simulink model "ALL_JP360_DBW_V6_5_1103"  (R2022a)
settings: Solver=FixedStepAuto  StartTime=0.0  StopTime=inf  FixedStep=0.01  RelTol=1e-3  EnableMultiTasking=on
model workspace (MAT data in the model file):
  g = 9.8
undefined symbols (not defined in the file or in its folder): canChannel, delta_v_p, IPM_Line_C0, IPM_Line_C1, IPM_Line_C2, IPM_Line_C3, M, M_p, MRR_ObjDistX, MRR_ObjDistY, MRR_ObjFusionCamID, MRR_ObjFusionSig, MRR_ObjID, MRR_ObjRelVelX, MRR_ObjRelVelY, MRR_ObjType, MRR_ObjUpdFlg, none, obj_vaild, untracktime, V, videoinput
libraries: canfdmsglib x230, canfdlib x76, slpidlib x24, simulink x18, dspstat3 x14, ctrlSharedLib x1, simulink_extras x1, imaqlib x1, realtime_pacer_lib x1, dspvision x1, visionsinks x1
(part 41 of 55)

== system ALL_JP360_DBW_V6_5_1103/MsgFromCAN/Subsystem1/Subsystem17 ==
  VR_ADCU_MRR_ObjHeader_0x680FromOutData : Inport
  Bus Selector1 : BusSelector  OutputSignals=IPM_ObjBlockCounter_18,IPM_ObjDistX_18,IPM_ObjDistY_18,IPM_ObjID_18,IPM_ObjRelAccelX_18,IPM_ObjRelAccelY_18,IPM_ObjRelVelX_18,IPM_ObjRelVelY_18,IPM_ObjType_18,IPM_Object_Age_18,IPM_Object_Existence_Probability_18,IPM_Object_Heading_18,IPM_Object_Height_18,IPM_Object_Length_18,IPM_Object_Motion_Status_18,IPM_Object_Width_18
  Data Type Conversion{1..2,4,6,16..27} (16 alike) : DataTypeConversion  OutDataTypeStr=single  SaturateOnIntegerOverflow=off  RndMeth=Floor
  Mux1 : Mux  Inputs=16
  Out2 : Outport
  wires:
  Bus Selector1/12 -> Data Type Conversion27/1  "<IPM_Object_Heading_18>"
  Bus Selector1/10 -> Data Type Conversion25/1  "<IPM_Object_Age_18>"
  Bus Selector1/11 -> Data Type Conversion26/1  "<IPM_Object_Existence_Probability_18>"
  Bus Selector1/9 -> Data Type Conversion24/1  "<IPM_ObjType_18>"
  Bus Selector1/7 -> Data Type Conversion22/1  "<IPM_ObjRelVelX_18>"
  Bus Selector1/5 -> Data Type Conversion20/1  "<IPM_ObjRelAccelX_18>"
  Bus Selector1/4 -> Data Type Conversion19/1  "<IPM_ObjID_18>"
  Bus Selector1/8 -> Data Type Conversion23/1  "<IPM_ObjRelVelY_18>"
  Bus Selector1/6 -> Data Type Conversion21/1  "<IPM_ObjRelAccelY_18>"
  Bus Selector1/3 -> Data Type Conversion18/1  "<IPM_ObjDistY_18>"
  Mux1/1 -> Out2/1
  Bus Selector1/2 -> Data Type Conversion17/1  "<IPM_ObjDistX_18>"
  VR_ADCU_MRR_ObjHeader_0x680FromOutData/1 -> Bus Selector1/1
  Bus Selector1/1 -> Data Type Conversion16/1  "<IPM_ObjBlockCounter_18>"
  Data Type Conversion27/1 -> Mux1/12
  Data Type Conversion26/1 -> Mux1/11
  Data Type Conversion21/1 -> Mux1/6
  Data Type Conversion23/1 -> Mux1/8
  Data Type Conversion25/1 -> Mux1/10
  Data Type Conversion19/1 -> Mux1/4
  Data Type Conversion20/1 -> Mux1/5
  Data Type Conversion22/1 -> Mux1/7
  Data Type Conversion24/1 -> Mux1/9
  Data Type Conversion16/1 -> Mux1/1
  Data Type Conversion18/1 -> Mux1/3
  Data Type Conversion17/1 -> Mux1/2
  Bus Selector1/13 -> Data Type Conversion1/1  "<IPM_Object_Height_18>"
  Bus Selector1/14 -> Data Type Conversion2/1  "<IPM_Object_Length_18>"
  Bus Selector1/15 -> Data Type Conversion4/1  "<IPM_Object_Motion_Status_18>"
  Bus Selector1/16 -> Data Type Conversion6/1  "<IPM_Object_Width_18>"
  Data Type Conversion1/1 -> Mux1/13
  Data Type Conversion2/1 -> Mux1/14
  Data Type Conversion4/1 -> Mux1/15
  Data Type Conversion6/1 -> Mux1/16

== system ALL_JP360_DBW_V6_5_1103/MsgFromCAN/Subsystem1/Subsystem18 ==
  VR_ADCU_MRR_ObjHeader_0x680FromOutData : Inport
  Bus Selector1 : BusSelector  OutputSignals=IPM_ObjBlockCounter_16,IPM_ObjDistX_16,IPM_ObjDistY_16,IPM_ObjID_16,IPM_ObjRelAccelX_16,IPM_ObjRelAccelY_16,IPM_ObjRelVelX_16,IPM_ObjRelVelY_16,IPM_ObjType_16,IPM_Object_Age_16,IPM_Object_Existence_Probability_16,IPM_Object_Heading_16,IPM_Object_Height_16,IPM_Object_Length_16,IPM_Object_Motion_Status_16,IPM_Object_Width_16
  Data Type Conversion{1..2,4,6,16..27} (16 alike) : DataTypeConversion  OutDataTypeStr=single  SaturateOnIntegerOverflow=off  RndMeth=Floor
  Mux1 : Mux  Inputs=16
  Out2 : Outport
  wires:
  Bus Selector1/12 -> Data Type Conversion27/1  "<IPM_Object_Heading_16>"
  Bus Selector1/10 -> Data Type Conversion25/1  "<IPM_Object_Age_16>"
  Bus Selector1/11 -> Data Type Conversion26/1  "<IPM_Object_Existence_Probability_16>"
  Bus Selector1/9 -> Data Type Conversion24/1  "<IPM_ObjType_16>"
  Bus Selector1/7 -> Data Type Conversion22/1  "<IPM_ObjRelVelX_16>"
  Bus Selector1/5 -> Data Type Conversion20/1  "<IPM_ObjRelAccelX_16>"
  Bus Selector1/4 -> Data Type Conversion19/1  "<IPM_ObjID_16>"
  Bus Selector1/8 -> Data Type Conversion23/1  "<IPM_ObjRelVelY_16>"
  Bus Selector1/6 -> Data Type Conversion21/1  "<IPM_ObjRelAccelY_16>"
  Bus Selector1/3 -> Data Type Conversion18/1  "<IPM_ObjDistY_16>"
  Mux1/1 -> Out2/1
  Bus Selector1/2 -> Data Type Conversion17/1  "<IPM_ObjDistX_16>"
  VR_ADCU_MRR_ObjHeader_0x680FromOutData/1 -> Bus Selector1/1
  Bus Selector1/1 -> Data Type Conversion16/1  "<IPM_ObjBlockCounter_16>"
  Data Type Conversion27/1 -> Mux1/12
  Data Type Conversion26/1 -> Mux1/11
  Data Type Conversion21/1 -> Mux1/6
  Data Type Conversion23/1 -> Mux1/8
  Data Type Conversion25/1 -> Mux1/10
  Data Type Conversion19/1 -> Mux1/4
  Data Type Conversion20/1 -> Mux1/5
  Data Type Conversion22/1 -> Mux1/7
  Data Type Conversion24/1 -> Mux1/9
  Data Type Conversion16/1 -> Mux1/1
  Data Type Conversion18/1 -> Mux1/3
  Data Type Conversion17/1 -> Mux1/2
  Bus Selector1/13 -> Data Type Conversion1/1  "<IPM_Object_Height_16>"
  Bus Selector1/14 -> Data Type Conversion2/1  "<IPM_Object_Length_16>"
  Bus Selector1/15 -> Data Type Conversion4/1  "<IPM_Object_Motion_Status_16>"
  Bus Selector1/16 -> Data Type Conversion6/1  "<IPM_Object_Width_16>"
  Data Type Conversion1/1 -> Mux1/13
  Data Type Conversion2/1 -> Mux1/14
  Data Type Conversion4/1 -> Mux1/15
  Data Type Conversion6/1 -> Mux1/16

== system ALL_JP360_DBW_V6_5_1103/MsgFromCAN/Subsystem1/Subsystem19 ==
  VR_ADCU_MRR_ObjHeader_0x680FromOutData : Inport
  Bus Selector1 : BusSelector  OutputSignals=IPM_ObjBlockCounter_19,IPM_ObjDistX_19,IPM_ObjDistY_19,IPM_ObjID_19,IPM_ObjRelAccelX_19,IPM_ObjRelAccelY_19,IPM_ObjRelVelX_19,IPM_ObjRelVelY_19,IPM_ObjType_19,IPM_Object_Age_19,IPM_Object_Existence_Probability_19,IPM_Object_Heading_19,IPM_Object_Height_19,IPM_Object_Length_19,IPM_Object_Motion_Status_19,IPM_Object_Width_19
  Data Type Conversion{1..2,4,6,16..27} (16 alike) : DataTypeConversion  OutDataTypeStr=single  SaturateOnIntegerOverflow=off  RndMeth=Floor
  Mux1 : Mux  Inputs=16
  Out2 : Outport
  wires:
  Data Type Conversion6/1 -> Mux1/16
  Data Type Conversion4/1 -> Mux1/15
  Data Type Conversion2/1 -> Mux1/14
  Data Type Conversion1/1 -> Mux1/13
  Bus Selector1/16 -> Data Type Conversion6/1  "<IPM_Object_Width_19>"
  Bus Selector1/15 -> Data Type Conversion4/1  "<IPM_Object_Motion_Status_19>"
  Bus Selector1/14 -> Data Type Conversion2/1  "<IPM_Object_Length_19>"
  Bus Selector1/13 -> Data Type Conversion1/1  "<IPM_Object_Height_19>"
  Data Type Conversion17/1 -> Mux1/2
  Data Type Conversion18/1 -> Mux1/3
  Data Type Conversion16/1 -> Mux1/1
  Data Type Conversion24/1 -> Mux1/9
  Data Type Conversion22/1 -> Mux1/7
  Data Type Conversion20/1 -> Mux1/5
  Data Type Conversion19/1 -> Mux1/4
  Data Type Conversion25/1 -> Mux1/10
  Data Type Conversion23/1 -> Mux1/8
  Data Type Conversion21/1 -> Mux1/6
  Data Type Conversion26/1 -> Mux1/11
  Data Type Conversion27/1 -> Mux1/12
  Bus Selector1/1 -> Data Type Conversion16/1  "<IPM_ObjBlockCounter_19>"
  VR_ADCU_MRR_ObjHeader_0x680FromOutData/1 -> Bus Selector1/1
  Bus Selector1/2 -> Data Type Conversion17/1  "<IPM_ObjDistX_19>"
  Mux1/1 -> Out2/1
  Bus Selector1/3 -> Data Type Conversion18/1  "<IPM_ObjDistY_19>"
  Bus Selector1/6 -> Data Type Conversion21/1  "<IPM_ObjRelAccelY_19>"
  Bus Selector1/8 -> Data Type Conversion23/1  "<IPM_ObjRelVelY_19>"
  Bus Selector1/4 -> Data Type Conversion19/1  "<IPM_ObjID_19>"
  Bus Selector1/5 -> Data Type Conversion20/1  "<IPM_ObjRelAccelX_19>"
  Bus Selector1/7 -> Data Type Conversion22/1  "<IPM_ObjRelVelX_19>"
  Bus Selector1/9 -> Data Type Conversion24/1  "<IPM_ObjType_19>"
  Bus Selector1/11 -> Data Type Conversion26/1  "<IPM_Object_Existence_Probability_19>"
  Bus Selector1/10 -> Data Type Conversion25/1  "<IPM_Object_Age_19>"
  Bus Selector1/12 -> Data Type Conversion27/1  "<IPM_Object_Heading_19>"

== system ALL_JP360_DBW_V6_5_1103/MsgFromCAN/Subsystem1/Subsystem2 ==
  VR_ADCU_MRR_ObjHeader_0x680FromOutData : Inport
  Bus Selector1 : BusSelector  OutputSignals=IPM_ObjBlockCounter_03,IPM_ObjDistX_03,IPM_ObjDistY_03,IPM_ObjID_03,IPM_ObjRelAccelX_03,IPM_ObjRelAccelY_03,IPM_ObjRelVelX_03,IPM_ObjRelVelY_03,IPM_ObjType_03,IPM_Object_Age_03,IPM_Object_Existence_Probability_03,IPM_Object_Heading_03,IPM_Object_Height_03,IPM_Object_Length_03,IPM_Object_Motion_Status_03,IPM_Object_Width_03
  Data Type Conversion{1..2,4,6,16..27} (16 alike) : DataTypeConversion  OutDataTypeStr=single  SaturateOnIntegerOverflow=off  RndMeth=Floor
  Mux1 : Mux  Inputs=16
  Out2 : Outport
  wires:
  Bus Selector1/12 -> Data Type Conversion27/1  "<IPM_Object_Heading_03>"
  Bus Selector1/10 -> Data Type Conversion25/1  "<IPM_Object_Age_03>"
  Bus Selector1/11 -> Data Type Conversion26/1  "<IPM_Object_Existence_Probability_03>"
  Bus Selector1/9 -> Data Type Conversion24/1  "<IPM_ObjType_03>"
  Bus Selector1/7 -> Data Type Conversion22/1  "<IPM_ObjRelVelX_03>"
  Bus Selector1/5 -> Data Type Conversion20/1  "<IPM_ObjRelAccelX_03>"
  Bus Selector1/4 -> Data Type Conversion19/1  "<IPM_ObjID_03>"
  Bus Selector1/8 -> Data Type Conversion23/1  "<IPM_ObjRelVelY_03>"
  Bus Selector1/6 -> Data Type Conversion21/1  "<IPM_ObjRelAccelY_03>"
  Bus Selector1/3 -> Data Type Conversion18/1  "<IPM_ObjDistY_03>"
  Mux1/1 -> Out2/1
  Bus Selector1/2 -> Data Type Conversion17/1  "<IPM_ObjDistX_03>"
  VR_ADCU_MRR_ObjHeader_0x680FromOutData/1 -> Bus Selector1/1
  Bus Selector1/1 -> Data Type Conversion16/1  "<IPM_ObjBlockCounter_03>"
  Data Type Conversion27/1 -> Mux1/12
  Data Type Conversion26/1 -> Mux1/11
  Data Type Conversion21/1 -> Mux1/6
  Data Type Conversion23/1 -> Mux1/8
  Data Type Conversion25/1 -> Mux1/10
  Data Type Conversion19/1 -> Mux1/4
  Data Type Conversion20/1 -> Mux1/5
  Data Type Conversion22/1 -> Mux1/7
  Data Type Conversion24/1 -> Mux1/9
  Data Type Conversion16/1 -> Mux1/1
  Data Type Conversion18/1 -> Mux1/3
  Data Type Conversion17/1 -> Mux1/2
  Bus Selector1/13 -> Data Type Conversion1/1  "<IPM_Object_Height_03>"
  Bus Selector1/14 -> Data Type Conversion2/1  "<IPM_Object_Length_03>"
  Bus Selector1/15 -> Data Type Conversion4/1  "<IPM_Object_Motion_Status_03>"
  Bus Selector1/16 -> Data Type Conversion6/1  "<IPM_Object_Width_03>"
  Data Type Conversion1/1 -> Mux1/13
  Data Type Conversion2/1 -> Mux1/14
  Data Type Conversion4/1 -> Mux1/15
  Data Type Conversion6/1 -> Mux1/16

== system ALL_JP360_DBW_V6_5_1103/MsgFromCAN/Subsystem1/Subsystem20 ==
  VR_ADCU_MRR_ObjHeader_0x680FromOutData : Inport
  Bus Selector1 : BusSelector  OutputSignals=IPM_ObjBlockCounter_20,IPM_ObjDistX_20,IPM_ObjDistY_20,IPM_ObjID_20,IPM_ObjRelAccelX_20,IPM_ObjRelAccelY_20,IPM_ObjRelVelX_20,IPM_ObjRelVelY_20,IPM_ObjType_20,IPM_Object_Age_20,IPM_Object_Existence_Probability_20,IPM_Object_Heading_20,IPM_Object_Height_20,IPM_Object_Length_20,IPM_Object_Motion_Status_20,IPM_Object_Width_20
  Data Type Conversion{1..2,4,6,16..27} (16 alike) : DataTypeConversion  OutDataTypeStr=single  SaturateOnIntegerOverflow=off  RndMeth=Floor
  Mux1 : Mux  Inputs=16
  Out2 : Outport
  wires:
  Bus Selector1/12 -> Data Type Conversion27/1  "<IPM_Object_Heading_20>"
  Bus Selector1/10 -> Data Type Conversion25/1  "<IPM_Object_Age_20>"
  Bus Selector1/11 -> Data Type Conversion26/1  "<IPM_Object_Existence_Probability_20>"
  Bus Selector1/9 -> Data Type Conversion24/1  "<IPM_ObjType_20>"
  Bus Selector1/7 -> Data Type Conversion22/1  "<IPM_ObjRelVelX_20>"
  Bus Selector1/5 -> Data Type Conversion20/1  "<IPM_ObjRelAccelX_20>"
  Bus Selector1/4 -> Data Type Conversion19/1  "<IPM_ObjID_20>"
  Bus Selector1/8 -> Data Type Conversion23/1  "<IPM_ObjRelVelY_20>"
  Bus Selector1/6 -> Data Type Conversion21/1  "<IPM_ObjRelAccelY_20>"
  Bus Selector1/3 -> Data Type Conversion18/1  "<IPM_ObjDistY_20>"
  Mux1/1 -> Out2/1
  Bus Selector1/2 -> Data Type Conversion17/1  "<IPM_ObjDistX_20>"
  VR_ADCU_MRR_ObjHeader_0x680FromOutData/1 -> Bus Selector1/1
  Bus Selector1/1 -> Data Type Conversion16/1  "<IPM_ObjBlockCounter_20>"
  Data Type Conversion27/1 -> Mux1/12
  Data Type Conversion26/1 -> Mux1/11
  Data Type Conversion21/1 -> Mux1/6
  Data Type Conversion23/1 -> Mux1/8
  Data Type Conversion25/1 -> Mux1/10
  Data Type Conversion19/1 -> Mux1/4
  Data Type Conversion20/1 -> Mux1/5
  Data Type Conversion22/1 -> Mux1/7
  Data Type Conversion24/1 -> Mux1/9
  Data Type Conversion16/1 -> Mux1/1
  Data Type Conversion18/1 -> Mux1/3
  Data Type Conversion17/1 -> Mux1/2
  Bus Selector1/13 -> Data Type Conversion1/1  "<IPM_Object_Height_20>"
  Bus Selector1/14 -> Data Type Conversion2/1  "<IPM_Object_Length_20>"
  Bus Selector1/15 -> Data Type Conversion4/1  "<IPM_Object_Motion_Status_20>"
  Bus Selector1/16 -> Data Type Conversion6/1  "<IPM_Object_Width_20>"
  Data Type Conversion1/1 -> Mux1/13
  Data Type Conversion2/1 -> Mux1/14
  Data Type Conversion4/1 -> Mux1/15
  Data Type Conversion6/1 -> Mux1/16

== system ALL_JP360_DBW_V6_5_1103/MsgFromCAN/Subsystem1/Subsystem3 ==
  VR_ADCU_MRR_ObjHeader_0x680FromOutData : Inport
  Bus Selector1 : BusSelector  OutputSignals=IPM_ObjBlockCounter_05,IPM_ObjDistX_05,IPM_ObjDistY_05,IPM_ObjID_05,IPM_ObjRelAccelX_05,IPM_ObjRelAccelY_05,IPM_ObjRelVelX_05,IPM_ObjRelVelY_05,IPM_ObjType_05,IPM_Object_Age_05,IPM_Object_Existence_Probability_05,IPM_Object_Heading_05,IPM_Object_Height_05,IPM_Object_Length_05,IPM_Object_Motion_Status_05,IPM_Object_Width_05
  Data Type Conversion{1..2,4,6,16..27} (16 alike) : DataTypeConversion  OutDataTypeStr=single  SaturateOnIntegerOverflow=off  RndMeth=Floor
  Mux1 : Mux  Inputs=16
  Out2 : Outport
  wires:
  Data Type Conversion6/1 -> Mux1/16
  Data Type Conversion4/1 -> Mux1/15
  Data Type Conversion2/1 -> Mux1/14
  Data Type Conversion1/1 -> Mux1/13
  Bus Selector1/16 -> Data Type Conversion6/1  "<IPM_Object_Width_05>"
  Bus Selector1/15 -> Data Type Conversion4/1  "<IPM_Object_Motion_Status_05>"
  Bus Selector1/14 -> Data Type Conversion2/1  "<IPM_Object_Length_05>"
  Bus Selector1/13 -> Data Type Conversion1/1  "<IPM_Object_Height_05>"
  Data Type Conversion17/1 -> Mux1/2
  Data Type Conversion18/1 -> Mux1/3
  Data Type Conversion16/1 -> Mux1/1
  Data Type Conversion24/1 -> Mux1/9
  Data Type Conversion22/1 -> Mux1/7
  Data Type Conversion20/1 -> Mux1/5
  Data Type Conversion19/1 -> Mux1/4
  Data Type Conversion25/1 -> Mux1/10
  Data Type Conversion23/1 -> Mux1/8
  Data Type Conversion21/1 -> Mux1/6
  Data Type Conversion26/1 -> Mux1/11
  Data Type Conversion27/1 -> Mux1/12
  Bus Selector1/1 -> Data Type Conversion16/1  "<IPM_ObjBlockCounter_05>"
  VR_ADCU_MRR_ObjHeader_0x680FromOutData/1 -> Bus Selector1/1
  Bus Selector1/2 -> Data Type Conversion17/1  "<IPM_ObjDistX_05>"
  Mux1/1 -> Out2/1
  Bus Selector1/3 -> Data Type Conversion18/1  "<IPM_ObjDistY_05>"
  Bus Selector1/6 -> Data Type Conversion21/1  "<IPM_ObjRelAccelY_05>"
  Bus Selector1/8 -> Data Type Conversion23/1  "<IPM_ObjRelVelY_05>"
  Bus Selector1/4 -> Data Type Conversion19/1  "<IPM_ObjID_05>"
  Bus Selector1/5 -> Data Type Conversion20/1  "<IPM_ObjRelAccelX_05>"
  Bus Selector1/7 -> Data Type Conversion22/1  "<IPM_ObjRelVelX_05>"
  Bus Selector1/9 -> Data Type Conversion24/1  "<IPM_ObjType_05>"
  Bus Selector1/11 -> Data Type Conversion26/1  "<IPM_Object_Existence_Probability_05>"
  Bus Selector1/10 -> Data Type Conversion25/1  "<IPM_Object_Age_05>"
  Bus Selector1/12 -> Data Type Conversion27/1  "<IPM_Object_Heading_05>"

== system ALL_JP360_DBW_V6_5_1103/MsgFromCAN/Subsystem1/Subsystem4 ==
  VR_ADCU_MRR_ObjHeader_0x680FromOutData : Inport
  Bus Selector1 : BusSelector  OutputSignals=IPM_ObjBlockCounter_06,IPM_ObjDistX_06,IPM_ObjDistY_06,IPM_ObjID_06,IPM_ObjRelAccelX_06,IPM_ObjRelAccelY_06,IPM_ObjRelVelX_06,IPM_ObjRelVelY_06,IPM_ObjType_06,IPM_Object_Age_06,IPM_Object_Existence_Probability_06,IPM_Object_Heading_06,IPM_Object_Height_06,IPM_Object_Length_06,IPM_Object_Motion_Status_06,IPM_Object_Width_06
  Data Type Conversion{1..2,4,6,16..27} (16 alike) : DataTypeConversion  OutDataTypeStr=single  SaturateOnIntegerOverflow=off  RndMeth=Floor
  Mux1 : Mux  Inputs=16
  Out2 : Outport
  wires:
  Bus Selector1/12 -> Data Type Conversion27/1  "<IPM_Object_Heading_06>"
  Bus Selector1/10 -> Data Type Conversion25/1  "<IPM_Object_Age_06>"
  Bus Selector1/11 -> Data Type Conversion26/1  "<IPM_Object_Existence_Probability_06>"
  Bus Selector1/9 -> Data Type Conversion24/1  "<IPM_ObjType_06>"
  Bus Selector1/7 -> Data Type Conversion22/1  "<IPM_ObjRelVelX_06>"
  Bus Selector1/5 -> Data Type Conversion20/1  "<IPM_ObjRelAccelX_06>"
  Bus Selector1/4 -> Data Type Conversion19/1  "<IPM_ObjID_06>"
  Bus Selector1/8 -> Data Type Conversion23/1  "<IPM_ObjRelVelY_06>"
  Bus Selector1/6 -> Data Type Conversion21/1  "<IPM_ObjRelAccelY_06>"
  Bus Selector1/3 -> Data Type Conversion18/1  "<IPM_ObjDistY_06>"
  Mux1/1 -> Out2/1
  Bus Selector1/2 -> Data Type Conversion17/1  "<IPM_ObjDistX_06>"
  VR_ADCU_MRR_ObjHeader_0x680FromOutData/1 -> Bus Selector1/1
  Bus Selector1/1 -> Data Type Conversion16/1  "<IPM_ObjBlockCounter_06>"
  Data Type Conversion27/1 -> Mux1/12
  Data Type Conversion26/1 -> Mux1/11
  Data Type Conversion21/1 -> Mux1/6
  Data Type Conversion23/1 -> Mux1/8
  Data Type Conversion25/1 -> Mux1/10
  Data Type Conversion19/1 -> Mux1/4
  Data Type Conversion20/1 -> Mux1/5
  Data Type Conversion22/1 -> Mux1/7
  Data Type Conversion24/1 -> Mux1/9
  Data Type Conversion16/1 -> Mux1/1
  Data Type Conversion18/1 -> Mux1/3
  Data Type Conversion17/1 -> Mux1/2
  Bus Selector1/13 -> Data Type Conversion1/1  "<IPM_Object_Height_06>"
  Bus Selector1/14 -> Data Type Conversion2/1  "<IPM_Object_Length_06>"
  Bus Selector1/15 -> Data Type Conversion4/1  "<IPM_Object_Motion_Status_06>"
  Bus Selector1/16 -> Data Type Conversion6/1  "<IPM_Object_Width_06>"
  Data Type Conversion1/1 -> Mux1/13
  Data Type Conversion2/1 -> Mux1/14
  Data Type Conversion4/1 -> Mux1/15
  Data Type Conversion6/1 -> Mux1/16

== system ALL_JP360_DBW_V6_5_1103/MsgFromCAN/Subsystem1/Subsystem5 ==
  VR_ADCU_MRR_ObjHeader_0x680FromOutData : Inport
  Bus Selector1 : BusSelector  OutputSignals=IPM_ObjBlockCounter_04,IPM_ObjDistX_04,IPM_ObjDistY_04,IPM_ObjID_04,IPM_ObjRelAccelX_04,IPM_ObjRelAccelY_04,IPM_ObjRelVelX_04,IPM_ObjRelVelY_04,IPM_ObjType_04,IPM_Object_Age_04,IPM_Object_Existence_Probability_04,IPM_Object_Heading_04,IPM_Object_Height_04,IPM_Object_Length_04,IPM_Object_Motion_Status_04,IPM_Object_Width_04
  Data Type Conversion{1..2,4,6,16..27} (16 alike) : DataTypeConversion  OutDataTypeStr=single  SaturateOnIntegerOverflow=off  RndMeth=Floor
  Mux1 : Mux  Inputs=16
  Out2 : Outport
  wires:
  Bus Selector1/12 -> Data Type Conversion27/1  "<IPM_Object_Heading_04>"
  Bus Selector1/10 -> Data Type Conversion25/1  "<IPM_Object_Age_04>"
  Bus Selector1/11 -> Data Type Conversion26/1  "<IPM_Object_Existence_Probability_04>"
  Bus Selector1/9 -> Data Type Conversion24/1  "<IPM_ObjType_04>"
  Bus Selector1/7 -> Data Type Conversion22/1  "<IPM_ObjRelVelX_04>"
  Bus Selector1/5 -> Data Type Conversion20/1  "<IPM_ObjRelAccelX_04>"
  Bus Selector1/4 -> Data Type Conversion19/1  "<IPM_ObjID_04>"
  Bus Selector1/8 -> Data Type Conversion23/1  "<IPM_ObjRelVelY_04>"
  Bus Selector1/6 -> Data Type Conversion21/1  "<IPM_ObjRelAccelY_04>"
  Bus Selector1/3 -> Data Type Conversion18/1  "<IPM_ObjDistY_04>"
  Mux1/1 -> Out2/1
  Bus Selector1/2 -> Data Type Conversion17/1  "<IPM_ObjDistX_04>"
  VR_ADCU_MRR_ObjHeader_0x680FromOutData/1 -> Bus Selector1/1
  Bus Selector1/1 -> Data Type Conversion16/1  "<IPM_ObjBlockCounter_04>"
  Data Type Conversion27/1 -> Mux1/12
  Data Type Conversion26/1 -> Mux1/11
  Data Type Conversion21/1 -> Mux1/6
  Data Type Conversion23/1 -> Mux1/8
  Data Type Conversion25/1 -> Mux1/10
  Data Type Conversion19/1 -> Mux1/4
  Data Type Conversion20/1 -> Mux1/5
  Data Type Conversion22/1 -> Mux1/7
  Data Type Conversion24/1 -> Mux1/9
  Data Type Conversion16/1 -> Mux1/1
  Data Type Conversion18/1 -> Mux1/3
  Data Type Conversion17/1 -> Mux1/2
  Bus Selector1/13 -> Data Type Conversion1/1  "<IPM_Object_Height_04>"
  Bus Selector1/14 -> Data Type Conversion2/1  "<IPM_Object_Length_04>"
  Bus Selector1/15 -> Data Type Conversion4/1  "<IPM_Object_Motion_Status_04>"
  Bus Selector1/16 -> Data Type Conversion6/1  "<IPM_Object_Width_04>"
  Data Type Conversion1/1 -> Mux1/13
  Data Type Conversion2/1 -> Mux1/14
  Data Type Conversion4/1 -> Mux1/15
  Data Type Conversion6/1 -> Mux1/16

== system ALL_JP360_DBW_V6_5_1103/MsgFromCAN/Subsystem1/Subsystem6 ==
  VR_ADCU_MRR_ObjHeader_0x680FromOutData : Inport
  Bus Selector1 : BusSelector  OutputSignals=IPM_ObjBlockCounter_08,IPM_ObjDistX_08,IPM_ObjDistY_08,IPM_ObjID_08,IPM_ObjRelAccelX_08,IPM_ObjRelAccelY_08,IPM_ObjRelVelX_08,IPM_ObjRelVelY_08,IPM_ObjType_08,IPM_Object_Age_08,IPM_Object_Existence_Probability_08,IPM_Object_Heading_08,IPM_Object_Height_08,IPM_Object_Length_08,IPM_Object_Motion_Status_08,IPM_Object_Width_08
  Data Type Conversion{1..2,4,6,16..27} (16 alike) : DataTypeConversion  OutDataTypeStr=single  SaturateOnIntegerOverflow=off  RndMeth=Floor
  Mux1 : Mux  Inputs=16
  Out2 : Outport
  wires:
  Data Type Conversion6/1 -> Mux1/16
  Data Type Conversion4/1 -> Mux1/15
  Data Type Conversion2/1 -> Mux1/14
  Data Type Conversion1/1 -> Mux1/13
  Bus Selector1/16 -> Data Type Conversion6/1  "<IPM_Object_Width_08>"
  Bus Selector1/15 -> Data Type Conversion4/1  "<IPM_Object_Motion_Status_08>"
  Bus Selector1/14 -> Data Type Conversion2/1  "<IPM_Object_Length_08>"
  Bus Selector1/13 -> Data Type Conversion1/1  "<IPM_Object_Height_08>"
  Data Type Conversion17/1 -> Mux1/2
  Data Type Conversion18/1 -> Mux1/3
  Data Type Conversion16/1 -> Mux1/1
  Data Type Conversion24/1 -> Mux1/9
  Data Type Conversion22/1 -> Mux1/7
  Data Type Conversion20/1 -> Mux1/5
  Data Type Conversion19/1 -> Mux1/4
  Data Type Conversion25/1 -> Mux1/10
  Data Type Conversion23/1 -> Mux1/8
  Data Type Conversion21/1 -> Mux1/6
  Data Type Conversion26/1 -> Mux1/11
  Data Type Conversion27/1 -> Mux1/12
  Bus Selector1/1 -> Data Type Conversion16/1  "<IPM_ObjBlockCounter_08>"
  VR_ADCU_MRR_ObjHeader_0x680FromOutData/1 -> Bus Selector1/1
  Bus Selector1/2 -> Data Type Conversion17/1  "<IPM_ObjDistX_08>"
  Mux1/1 -> Out2/1
  Bus Selector1/3 -> Data Type Conversion18/1  "<IPM_ObjDistY_08>"
  Bus Selector1/6 -> Data Type Conversion21/1  "<IPM_ObjRelAccelY_08>"
  Bus Selector1/8 -> Data Type Conversion23/1  "<IPM_ObjRelVelY_08>"
  Bus Selector1/4 -> Data Type Conversion19/1  "<IPM_ObjID_08>"
  Bus Selector1/5 -> Data Type Conversion20/1  "<IPM_ObjRelAccelX_08>"
  Bus Selector1/7 -> Data Type Conversion22/1  "<IPM_ObjRelVelX_08>"
  Bus Selector1/9 -> Data Type Conversion24/1  "<IPM_ObjType_08>"
  Bus Selector1/11 -> Data Type Conversion26/1  "<IPM_Object_Existence_Probability_08>"
  Bus Selector1/10 -> Data Type Conversion25/1  "<IPM_Object_Age_08>"
  Bus Selector1/12 -> Data Type Conversion27/1  "<IPM_Object_Heading_08>"

== system ALL_JP360_DBW_V6_5_1103/MsgFromCAN/Subsystem1/Subsystem7 ==
  VR_ADCU_MRR_ObjHeader_0x680FromOutData : Inport
  Bus Selector1 : BusSelector  OutputSignals=IPM_ObjBlockCounter_01,IPM_ObjDistX_01,IPM_ObjDistY_01,IPM_ObjID_01,IPM_ObjRelAccelX_01,IPM_ObjRelAccelY_01,IPM_ObjRelVelX_01,IPM_ObjRelVelY_01,IPM_ObjType_01,IPM_Object_Age_01,IPM_Object_Existence_Probability_01,IPM_Object_Heading_01,IPM_Object_Height_01,IPM_Object_Length_01,IPM_Object_Motion_Status_01,IPM_Object_Width_01
  Data Type Conversion{1..2,4,6,16..27} (16 alike) : DataTypeConversion  OutDataTypeStr=single  SaturateOnIntegerOverflow=off  RndMeth=Floor
  Mux1 : Mux  Inputs=16
  Out2 : Outport
  wires:
  Bus Selector1/12 -> Data Type Conversion27/1  "<IPM_Object_Heading_01>"
  Bus Selector1/10 -> Data Type Conversion25/1  "<IPM_Object_Age_01>"
  Bus Selector1/11 -> Data Type Conversion26/1  "<IPM_Object_Existence_Probability_01>"
  Bus Selector1/9 -> Data Type Conversion24/1  "<IPM_ObjType_01>"
  Bus Selector1/7 -> Data Type Conversion22/1  "<IPM_ObjRelVelX_01>"
  Bus Selector1/5 -> Data Type Conversion20/1  "<IPM_ObjRelAccelX_01>"
  Bus Selector1/4 -> Data Type Conversion19/1  "<IPM_ObjID_01>"
  Bus Selector1/8 -> Data Type Conversion23/1  "<IPM_ObjRelVelY_01>"
  Bus Selector1/6 -> Data Type Conversion21/1  "<IPM_ObjRelAccelY_01>"
  Bus Selector1/3 -> Data Type Conversion18/1  "<IPM_ObjDistY_01>"
  Mux1/1 -> Out2/1
  Bus Selector1/2 -> Data Type Conversion17/1  "<IPM_ObjDistX_01>"
  VR_ADCU_MRR_ObjHeader_0x680FromOutData/1 -> Bus Selector1/1
  Bus Selector1/1 -> Data Type Conversion16/1  "<IPM_ObjBlockCounter_01>"
  Data Type Conversion27/1 -> Mux1/12
  Data Type Conversion26/1 -> Mux1/11
  Data Type Conversion21/1 -> Mux1/6
  Data Type Conversion23/1 -> Mux1/8
  Data Type Conversion25/1 -> Mux1/10
  Data Type Conversion19/1 -> Mux1/4
  Data Type Conversion20/1 -> Mux1/5
  Data Type Conversion22/1 -> Mux1/7
  Data Type Conversion24/1 -> Mux1/9
  Data Type Conversion16/1 -> Mux1/1
  Data Type Conversion18/1 -> Mux1/3
  Data Type Conversion17/1 -> Mux1/2
  Bus Selector1/13 -> Data Type Conversion1/1  "<IPM_Object_Height_01>"
  Bus Selector1/14 -> Data Type Conversion2/1  "<IPM_Object_Length_01>"
  Bus Selector1/15 -> Data Type Conversion4/1  "<IPM_Object_Motion_Status_01>"
  Bus Selector1/16 -> Data Type Conversion6/1  "<IPM_Object_Width_01>"
  Data Type Conversion1/1 -> Mux1/13
  Data Type Conversion2/1 -> Mux1/14
  Data Type Conversion4/1 -> Mux1/15
  Data Type Conversion6/1 -> Mux1/16

== system ALL_JP360_DBW_V6_5_1103/MsgFromCAN/Subsystem1/Subsystem8 ==
  VR_ADCU_MRR_ObjHeader_0x680FromOutData : Inport
  Bus Selector1 : BusSelector  OutputSignals=IPM_ObjBlockCounter_09,IPM_ObjDistX_09,IPM_ObjDistY_09,IPM_ObjID_09,IPM_ObjRelAccelX_09,IPM_ObjRelAccelY_09,IPM_ObjRelVelX_09,IPM_ObjRelVelY_09,IPM_ObjType_09,IPM_Object_Age_09,IPM_Object_Existence_Probability_09,IPM_Object_Heading_09,IPM_Object_Height_09,IPM_Object_Length_09,IPM_Object_Motion_Status_09,IPM_Object_Width_09
  Data Type Conversion{1..2,4,6,16..27} (16 alike) : DataTypeConversion  OutDataTypeStr=single  SaturateOnIntegerOverflow=off  RndMeth=Floor
  Mux1 : Mux  Inputs=16
  Out2 : Outport
  wires:
  Bus Selector1/12 -> Data Type Conversion27/1  "<IPM_Object_Heading_09>"
  Bus Selector1/10 -> Data Type Conversion25/1  "<IPM_Object_Age_09>"
  Bus Selector1/11 -> Data Type Conversion26/1  "<IPM_Object_Existence_Probability_09>"
  Bus Selector1/9 -> Data Type Conversion24/1  "<IPM_ObjType_09>"
  Bus Selector1/7 -> Data Type Conversion22/1  "<IPM_ObjRelVelX_09>"
  Bus Selector1/5 -> Data Type Conversion20/1  "<IPM_ObjRelAccelX_09>"
  Bus Selector1/4 -> Data Type Conversion19/1  "<IPM_ObjID_09>"
  Bus Selector1/8 -> Data Type Conversion23/1  "<IPM_ObjRelVelY_09>"
  Bus Selector1/6 -> Data Type Conversion21/1  "<IPM_ObjRelAccelY_09>"
  Bus Selector1/3 -> Data Type Conversion18/1  "<IPM_ObjDistY_09>"
  Mux1/1 -> Out2/1
  Bus Selector1/2 -> Data Type Conversion17/1  "<IPM_ObjDistX_09>"
  VR_ADCU_MRR_ObjHeader_0x680FromOutData/1 -> Bus Selector1/1
  Bus Selector1/1 -> Data Type Conversion16/1  "<IPM_ObjBlockCounter_09>"
  Data Type Conversion27/1 -> Mux1/12
  Data Type Conversion26/1 -> Mux1/11
  Data Type Conversion21/1 -> Mux1/6
  Data Type Conversion23/1 -> Mux1/8
  Data Type Conversion25/1 -> Mux1/10
  Data Type Conversion19/1 -> Mux1/4
  Data Type Conversion20/1 -> Mux1/5
  Data Type Conversion22/1 -> Mux1/7
  Data Type Conversion24/1 -> Mux1/9
  Data Type Conversion16/1 -> Mux1/1
  Data Type Conversion18/1 -> Mux1/3
  Data Type Conversion17/1 -> Mux1/2
  Bus Selector1/13 -> Data Type Conversion1/1  "<IPM_Object_Height_09>"
  Bus Selector1/14 -> Data Type Conversion2/1  "<IPM_Object_Length_09>"
  Bus Selector1/15 -> Data Type Conversion4/1  "<IPM_Object_Motion_Status_09>"
  Bus Selector1/16 -> Data Type Conversion6/1  "<IPM_Object_Width_09>"
  Data Type Conversion1/1 -> Mux1/13
  Data Type Conversion2/1 -> Mux1/14
  Data Type Conversion4/1 -> Mux1/15
  Data Type Conversion6/1 -> Mux1/16

== system ALL_JP360_DBW_V6_5_1103/MsgFromCAN/Subsystem1/Subsystem9 ==
  VR_ADCU_MRR_ObjHeader_0x680FromOutData : Inport
  Bus Selector1 : BusSelector  OutputSignals=IPM_ObjBlockCounter_07,IPM_ObjDistX_07,IPM_ObjDistY_07,IPM_ObjID_07,IPM_ObjRelAccelX_07,IPM_ObjRelAccelY_07,IPM_ObjRelVelX_07,IPM_ObjRelVelY_07,IPM_ObjType_07,IPM_Object_Age_07,IPM_Object_Existence_Probability_07,IPM_Object_Heading_07,IPM_Object_Height_07,IPM_Object_Length_07,IPM_Object_Motion_Status_07,IPM_Object_Width_07
  Data Type Conversion{1..2,4,6,16..27} (16 alike) : DataTypeConversion  OutDataTypeStr=single  SaturateOnIntegerOverflow=off  RndMeth=Floor
  Mux1 : Mux  Inputs=16
  Out2 : Outport
  wires:
  Bus Selector1/12 -> Data Type Conversion27/1  "<IPM_Object_Heading_07>"
  Bus Selector1/10 -> Data Type Conversion25/1  "<IPM_Object_Age_07>"
  Bus Selector1/11 -> Data Type Conversion26/1  "<IPM_Object_Existence_Probability_07>"
  Bus Selector1/9 -> Data Type Conversion24/1  "<IPM_ObjType_07>"
  Bus Selector1/7 -> Data Type Conversion22/1  "<IPM_ObjRelVelX_07>"
  Bus Selector1/5 -> Data Type Conversion20/1  "<IPM_ObjRelAccelX_07>"
  Bus Selector1/4 -> Data Type Conversion19/1  "<IPM_ObjID_07>"
  Bus Selector1/8 -> Data Type Conversion23/1  "<IPM_ObjRelVelY_07>"
  Bus Selector1/6 -> Data Type Conversion21/1  "<IPM_ObjRelAccelY_07>"
  Bus Selector1/3 -> Data Type Conversion18/1  "<IPM_ObjDistY_07>"
  Mux1/1 -> Out2/1
  Bus Selector1/2 -> Data Type Conversion17/1  "<IPM_ObjDistX_07>"
  VR_ADCU_MRR_ObjHeader_0x680FromOutData/1 -> Bus Selector1/1
  Bus Selector1/1 -> Data Type Conversion16/1  "<IPM_ObjBlockCounter_07>"
  Data Type Conversion27/1 -> Mux1/12
  Data Type Conversion26/1 -> Mux1/11
  Data Type Conversion21/1 -> Mux1/6
  Data Type Conversion23/1 -> Mux1/8
  Data Type Conversion25/1 -> Mux1/10
  Data Type Conversion19/1 -> Mux1/4
  Data Type Conversion20/1 -> Mux1/5
  Data Type Conversion22/1 -> Mux1/7
  Data Type Conversion24/1 -> Mux1/9
  Data Type Conversion16/1 -> Mux1/1
  Data Type Conversion18/1 -> Mux1/3
  Data Type Conversion17/1 -> Mux1/2
  Bus Selector1/13 -> Data Type Conversion1/1  "<IPM_Object_Height_07>"
  Bus Selector1/14 -> Data Type Conversion2/1  "<IPM_Object_Length_07>"
  Bus Selector1/15 -> Data Type Conversion4/1  "<IPM_Object_Motion_Status_07>"
  Bus Selector1/16 -> Data Type Conversion6/1  "<IPM_Object_Width_07>"
  Data Type Conversion1/1 -> Mux1/13
  Data Type Conversion2/1 -> Mux1/14
  Data Type Conversion4/1 -> Mux1/15
  Data Type Conversion6/1 -> Mux1/16

== system ALL_JP360_DBW_V6_5_1103/MsgFromCAN/VR_ADCU_MsgFromCAN/VR_ADCU_IPM_0x345 ==
  VR_ADCU_IPM_0x345FromInData : Inport  OutDataTypeStr=Bus:CAN_FD_MESSAGE_BUS
  Bus Creator : BusCreator  Inputs=21  OutDataTypeStr=Bus:VR_ADCU_IPM_0x345  NonVirtualBus=on
  CAN FD Unpack : canfdmsglib/CAN FD Unpack  CANdbFile=HiFire_T360_P789_1R1V_Pri_Matrix_CAN_V2.3_20220810.dbc  MsgList=(none)  MsgName=IPM_0x345  ProtocolMode=CAN FD  MsgIDType=Standard (11-bit identifier)  MsgIdentifier=837  MsgLength=8  SignalInfo={'Checksum_0x245','56','8','BE','unsigned','Standard','0','1','0','0','255';'IPM_ADAS_Alerts','43','3','BE','unsigned','Standard','0','1','0','0','7';'IPM_IHC_HighbeamReq','55','1','BE','unsigned','Standard','0','1','0','0','1';'IPM_IHC_Status','40','3','BE','unsigned','Standard','0','1','0','0','7';'IPM_LDWWarningType','52','2','BE','unsigned','Standard','0','1','0','0','3';'IPM_LineAssitType','22','3','BE','unsigned','Standard','0','1','0','0','7';'IPM_LineAssit_HandsonReq','54','1','BE','unsigned','Standard','0','1','0','0','1';'IPM_LineAssit_LeftVisualization','18','2','BE','unsigned','Standard','0','1','0','0','3';'IPM_LineAssit_RightVisualization','20','2','BE','unsigned','Standard','0','1','0','0','3';'IPM_LineAssit_Sensitivity','16','1','BE','unsigned','Standard','0','1','0','0','1';'IPM_LineAssit_Status','29','3','BE','unsigned','Standard','0','1','0','0','7';'IPM_LineAssit_TorqueReq','13','11','BE','unsigned','Standard','0','0.01','-10.24','-10.24','10.22';'IPM_LineAssit_TorqueReqStatus','10','2','BE','unsigned','Standard','0','1','0','0','3';'IPM_LineAssit_TorqueValidity','12','1','BE','unsigned','Standard','0','1','0','0','1';'IPM_LineAssit_WarningAudio','17','1','BE','unsigned','Standard','0','1','0','0','1';'IPM_LineAssit_WarningVibration','9','1','BE','unsigned','Standard','0','1','0','0','1';'IPM_SLA_Spdlimit','32','8','BE','unsigned','Standard','0','1','0','0','255';'IPM_SLA_SpdlimitUnits','24','2','BE','unsigned','Standard','0','1','0','0','3';'IPM_SLA_Status','26','3','BE','unsigned','Standard','0','1','0','0','7';'IPM_TJAICA_Status','47','1','BE','unsigned','Standard','0','1','0','0','1';'RollingCounter_0x245','48','4','BE','unsigned','Standard','0','1','0','0','15'}  IDPort=off  TimestampPort=off  ErrorPort=off  RemotePort=off  LengthPort=off  StatusPort=off  BRSPort=off  ESIPort=off  DLCPort=off  ApplyMinMax=off
      settings: SourceProductBaseCode=ME,XP,VN  DataFormat=CANdb specified signals
  Data Type Conversion1 : DataTypeConversion  OutDataTypeStr=uint8  SaturateOnIntegerOverflow=off  RndMeth=Floor
  Data Type Conversion{3,7,10,14..16,20} (7 alike) : DataTypeConversion  OutDataTypeStr=boolean  SaturateOnIntegerOverflow=off  RndMeth=Floor
  Data Type Conversion{2,4..6,8..9,11,13,18..19,21} (11 alike) : DataTypeConversion  OutDataTypeStr=int8  SaturateOnIntegerOverflow=off  RndMeth=Floor
  Data Type Conversion12 : DataTypeConversion  OutDataTypeStr=single  SaturateOnIntegerOverflow=off  RndMeth=Floor
  Data Type Conversion17 : DataTypeConversion  OutDataTypeStr=uint8  SaturateOnIntegerOverflow=off  RndMeth=Floor
  VR_ADCU_IPM_0x345FromOutData : Outport  OutDataTypeStr=Bus:VR_ADCU_IPM_0x345
  wires:
  CAN FD Unpack/1 -> Data Type Conversion1/1
  CAN FD Unpack/2 -> Data Type Conversion2/1
  CAN FD Unpack/3 -> Data Type Conversion3/1
  CAN FD Unpack/4 -> Data Type Conversion4/1
  CAN FD Unpack/5 -> Data Type Conversion5/1
  CAN FD Unpack/6 -> Data Type Conversion6/1
  CAN FD Unpack/7 -> Data Type Conversion7/1
  CAN FD Unpack/8 -> Data Type Conversion8/1
  CAN FD Unpack/9 -> Data Type Conversion9/1
  CAN FD Unpack/10 -> Data Type Conversion10/1
  CAN FD Unpack/11 -> Data Type Conversion11/1
  CAN FD Unpack/12 -> Data Type Conversion12/1
  CAN FD Unpack/13 -> Data Type Conversion13/1
  CAN FD Unpack/14 -> Data Type Conversion14/1
  CAN FD Unpack/15 -> Data Type Conversion15/1
  CAN FD Unpack/16 -> Data Type Conversion16/1
  CAN FD Unpack/17 -> Data Type Conversion17/1
  CAN FD Unpack/18 -> Data Type Conversion18/1
  CAN FD Unpack/19 -> Data Type Conversion19/1
  CAN FD Unpack/20 -> Data Type Conversion20/1
  CAN FD Unpack/21 -> Data Type Conversion21/1
  Data Type Conversion1/1 -> Bus Creator/1  "Checksum_0x245"
  Data Type Conversion2/1 -> Bus Creator/2  "IPM_ADAS_Alerts"
  Data Type Conversion3/1 -> Bus Creator/3  "IPM_IHC_HighbeamReq"
  Data Type Conversion4/1 -> Bus Creator/4  "IPM_IHC_Status"
  Data Type Conversion5/1 -> Bus Creator/5  "IPM_LDWWarningType"
  Data Type Conversion6/1 -> Bus Creator/6  "IPM_LineAssitType"
  Data Type Conversion7/1 -> Bus Creator/7  "IPM_LineAssit_HandsonReq"
  Data Type Conversion8/1 -> Bus Creator/8  "IPM_LineAssit_LeftVisualization"
  Data Type Conversion9/1 -> Bus Creator/9  "IPM_LineAssit_RightVisualization"
  Data Type Conversion10/1 -> Bus Creator/10  "IPM_LineAssit_Sensitivity"
  Data Type Conversion11/1 -> Bus Creator/11  "IPM_LineAssit_Status"
  Data Type Conversion12/1 -> Bus Creator/12  "IPM_LineAssit_TorqueReq"
  Data Type Conversion13/1 -> Bus Creator/13  "IPM_LineAssit_TorqueReqStatus"
  Data Type Conversion14/1 -> Bus Creator/14  "IPM_LineAssit_TorqueValidity"
  Data Type Conversion15/1 -> Bus Creator/15  "IPM_LineAssit_WarningAudio"
  Data Type Conversion16/1 -> Bus Creator/16  "IPM_LineAssit_WarningVibration"
  Data Type Conversion17/1 -> Bus Creator/17  "IPM_SLA_Spdlimit"
  Data Type Conversion18/1 -> Bus Creator/18  "IPM_SLA_SpdlimitUnits"
  Data Type Conversion19/1 -> Bus Creator/19  "IPM_SLA_Status"
  Data Type Conversion20/1 -> Bus Creator/20  "IPM_TJAICA_Status"
  Data Type Conversion21/1 -> Bus Creator/21  "RollingCounter_0x245"
  Bus Creator/1 -> VR_ADCU_IPM_0x345FromOutData/1  "VR_ADCU_IPM_0x345FromOutData"
  VR_ADCU_IPM_0x345FromInData/1 -> CAN FD Unpack/1  "VR_ADCU_IPM_0x345FromInData"

== system ALL_JP360_DBW_V6_5_1103/MsgFromCAN/VR_ADCU_MsgFromCAN/VR_ADCU_IPM_0x347 ==
  VR_ADCU_IPM_0x347FromInData : Inport  OutDataTypeStr=Bus:CAN_FD_MESSAGE_BUS
  Bus Creator : BusCreator  Inputs=7  OutDataTypeStr=Bus:VR_ADCU_IPM_0x347  NonVirtualBus=on
  CAN FD Unpack : canfdmsglib/CAN FD Unpack  CANdbFile=HiFire_T360_P789_1R1V_Pri_Matrix_CAN_V2.3_20220810.dbc  MsgList=(none)  MsgName=IPM_0x347  ProtocolMode=CAN FD  MsgIDType=Standard (11-bit identifier)  MsgIdentifier=839  MsgLength=8  SignalInfo={'Checksum_0x247','56','8','BE','unsigned','Standard','0','1','0','0','255';'IPM_DCLCSts','5','3','BE','unsigned','Standard','0','1','0','0','7';'IPM_DCLC_manualfeedback','14','4','BE','unsigned','Standard','0','1','0','0','7';'IPM_ELKSts','2','3','BE','unsigned','Standard','0','1','0','0','7';'IPM_Traffic_Sign_Dis','16','8','BE','unsigned','Standard','0','1','0','0','255';'IPM_TurnIndicatorReq','12','2','BE','unsigned','Standard','0','1','0','0','3';'RollingCounter_0x247','48','4','BE','unsigned','Standard','0','1','0','0','15'}  IDPort=off  TimestampPort=off  ErrorPort=off  RemotePort=off  LengthPort=off  StatusPort=off  BRSPort=off  ESIPort=off  DLCPort=off  ApplyMinMax=off
      settings: SourceProductBaseCode=ME,XP,VN  DataFormat=CANdb specified signals
  Data Type Conversion1 : DataTypeConversion  OutDataTypeStr=uint8  SaturateOnIntegerOverflow=off  RndMeth=Floor
  Data Type Conversion{2..4,6..7} (5 alike) : DataTypeConversion  OutDataTypeStr=int8  SaturateOnIntegerOverflow=off  RndMeth=Floor
  Data Type Conversion5 : DataTypeConversion  OutDataTypeStr=uint8  SaturateOnIntegerOverflow=off  RndMeth=Floor
  VR_ADCU_IPM_0x347FromOutData : Outport  OutDataTypeStr=Bus:VR_ADCU_IPM_0x347
  wires:
  CAN FD Unpack/1 -> Data Type Conversion1/1
  CAN FD Unpack/2 -> Data Type Conversion2/1
  CAN FD Unpack/3 -> Data Type Conversion3/1
  CAN FD Unpack/4 -> Data Type Conversion4/1
  CAN FD Unpack/5 -> Data Type Conversion5/1
  CAN FD Unpack/6 -> Data Type Conversion6/1
  CAN FD Unpack/7 -> Data Type Conversion7/1
  Data Type Conversion1/1 -> Bus Creator/1  "Checksum_0x247"
  Data Type Conversion2/1 -> Bus Creator/2  "IPM_DCLCSts"
  Data Type Conversion3/1 -> Bus Creator/3  "IPM_DCLC_manualfeedback"
  Data Type Conversion4/1 -> Bus Creator/4  "IPM_ELKSts"
  Data Type Conversion5/1 -> Bus Creator/5  "IPM_Traffic_Sign_Dis"
  Data Type Conversion6/1 -> Bus Creator/6  "IPM_TurnIndicatorReq"
  Data Type Conversion7/1 -> Bus Creator/7  "RollingCounter_0x247"
  Bus Creator/1 -> VR_ADCU_IPM_0x347FromOutData/1  "VR_ADCU_IPM_0x347FromOutData"
  VR_ADCU_IPM_0x347FromInData/1 -> CAN FD Unpack/1  "VR_ADCU_IPM_0x347FromInData"

== system ALL_JP360_DBW_V6_5_1103/MsgFromCAN/VR_ADCU_MsgFromCAN/VR_ADCU_IPM_LeftLine_0x378 ==
  VR_ADCU_IPM_LeftLine_0x378FromInData : Inport  OutDataTypeStr=Bus:CAN_FD_MESSAGE_BUS
  Bus Creator : BusCreator  Inputs=6  OutDataTypeStr=Bus:VR_ADCU_IPM_LeftLine_0x378  NonVirtualBus=on
  CAN FD Unpack : canfdmsglib/CAN FD Unpack  CANdbFile=HiFire_T360_P789_1R1V_Pri_Matrix_CAN_V2.3_20220810.dbc  MsgList=(none)  MsgName=IPM_LeftLine_0x378  ProtocolMode=CAN FD  MsgIDType=Standard (11-bit identifier)  MsgIdentifier=888  MsgLength=8  SignalInfo={'IPM_LedtLine_dx_start','0','8','BE','unsigned','Standard','0','0.25','0','0','63.75';'IPM_LeftLine_dx_lookhead','27','9','BE','unsigned','Standard','0','0.25','0','0','127.75';'IPM_LeftLine_dy','20','12','BE','unsigned','Standard','0','0.0039062','-8','-8','7.9961';'IPM_LeftLine_hor_curvature_alteration','58','10','BE','unsigned','Standard','0','0.0001','-0.015','-0.015','0.0873';'IPM_LeftLine_hor_curve','33','10','BE','unsigned','Standard','0','0.0001','-0.015','-0.015','0.0873';'IPM_LeftLine_yawangle','52','12','BE','unsigned','Standard','0','0.00048828','-1','-1','0.99951'}  IDPort=off  TimestampPort=off  ErrorPort=off  RemotePort=off  LengthPort=off  StatusPort=off  BRSPort=off  ESIPort=off  DLCPort=off  ApplyMinMax=off
      settings: SourceProductBaseCode=ME,XP,VN  DataFormat=CANdb specified signals
  Data Type Conversion{1..6} (6 alike) : DataTypeConversion  OutDataTypeStr=single  SaturateOnIntegerOverflow=off  RndMeth=Floor
  VR_ADCU_IPM_LeftLine_0x378FromOutData : Outport  OutDataTypeStr=Bus:VR_ADCU_IPM_LeftLine_0x378
  wires:
  CAN FD Unpack/1 -> Data Type Conversion1/1
  CAN FD Unpack/2 -> Data Type Conversion2/1
  CAN FD Unpack/3 -> Data Type Conversion3/1
  CAN FD Unpack/4 -> Data Type Conversion4/1
  CAN FD Unpack/5 -> Data Type Conversion5/1
  CAN FD Unpack/6 -> Data Type Conversion6/1
  Data Type Conversion1/1 -> Bus Creator/1  "IPM_LedtLine_dx_start"
  Data Type Conversion2/1 -> Bus Creator/2  "IPM_LeftLine_dx_lookhead"
  Data Type Conversion3/1 -> Bus Creator/3  "IPM_LeftLine_dy"
  Data Type Conversion4/1 -> Bus Creator/4  "IPM_LeftLine_hor_curvature_alteration"
  Data Type Conversion5/1 -> Bus Creator/5  "IPM_LeftLine_hor_curve"
  Data Type Conversion6/1 -> Bus Creator/6  "IPM_LeftLine_yawangle"
  Bus Creator/1 -> VR_ADCU_IPM_LeftLine_0x378FromOutData/1  "VR_ADCU_IPM_LeftLine_0x378FromOutData"
  VR_ADCU_IPM_LeftLine_0x378FromInData/1 -> CAN FD Unpack/1  "VR_ADCU_IPM_LeftLine_0x378FromInData"

== system ALL_JP360_DBW_V6_5_1103/MsgFromCAN/VR_ADCU_MsgFromCAN/VR_ADCU_IPM_LeftLine_0x380 ==
  VR_ADCU_IPM_LeftLine_0x380FromInData : Inport  OutDataTypeStr=Bus:CAN_FD_MESSAGE_BUS
  Bus Creator : BusCreator  Inputs=9  OutDataTypeStr=Bus:VR_ADCU_IPM_LeftLine_0x380  NonVirtualBus=on
  CAN FD Unpack : canfdmsglib/CAN FD Unpack  CANdbFile=HiFire_T360_P789_1R1V_Pri_Matrix_CAN_V2.3_20220810.dbc  MsgList=(none)  MsgName=IPM_LeftLine_0x380  ProtocolMode=CAN FD  MsgIDType=Standard (11-bit identifier)  MsgIdentifier=896  MsgLength=8  SignalInfo={'IPM_LeftLeftLine_Color','13','3','BE','unsigned','Standard','0','1','0','0','7';'IPM_LeftLeftLine_Type','10','3','BE','unsigned','Standard','0','1','0','0','7';'IPM_LeftLeftLine_curvature_alteration','56','12','BE','unsigned','Standard','0','0.0001','-0.015','-0.015','0.0873';'IPM_LeftLeftLine_dy','28','12','BE','unsigned','Standard','0','0.0039062','-8','-8','7.9961';'IPM_LeftLeftLine_hor_curve','33','10','BE','unsigned','Standard','0','0.0001','-0.015','-0.015','0.0873';'IPM_LeftLeftLine_yawangle','52','12','BE','unsigned','Standard','0','0.00048828','-1','-1','0.99951';'IPM_LeftLine_Color','5','3','BE','unsigned','Standard','0','1','0','0','7';'IPM_LeftLine_Type','2','3','BE','unsigned','Standard','0','1','0','0','7';'IPM_LineAssit_LeftLeftVisualization','0','2','BE','unsigned','Standard','0','1','0','0','3'}  IDPort=off  TimestampPort=off  ErrorPort=off  RemotePort=off  LengthPort=off  StatusPort=off  BRSPort=off  ESIPort=off  DLCPort=off  ApplyMinMax=off
      settings: SourceProductBaseCode=ME,XP,VN  DataFormat=CANdb specified signals
  Data Type Conversion{1..2,7..9} (5 alike) : DataTypeConversion  OutDataTypeStr=int8  SaturateOnIntegerOverflow=off  RndMeth=Floor
  Data Type Conversion{3..6} (4 alike) : DataTypeConversion  OutDataTypeStr=single  SaturateOnIntegerOverflow=off  RndMeth=Floor
  VR_ADCU_IPM_LeftLine_0x380FromOutData : Outport  OutDataTypeStr=Bus:VR_ADCU_IPM_LeftLine_0x380
  wires:
  CAN FD Unpack/1 -> Data Type Conversion1/1
  CAN FD Unpack/2 -> Data Type Conversion2/1
  CAN FD Unpack/3 -> Data Type Conversion3/1
  CAN FD Unpack/4 -> Data Type Conversion4/1
  CAN FD Unpack/5 -> Data Type Conversion5/1
  CAN FD Unpack/6 -> Data Type Conversion6/1
  CAN FD Unpack/7 -> Data Type Conversion7/1
  CAN FD Unpack/8 -> Data Type Conversion8/1
  CAN FD Unpack/9 -> Data Type Conversion9/1
  Data Type Conversion1/1 -> Bus Creator/1  "IPM_LeftLeftLine_Color"
  Data Type Conversion2/1 -> Bus Creator/2  "IPM_LeftLeftLine_Type"
  Data Type Conversion3/1 -> Bus Creator/3  "IPM_LeftLeftLine_curvature_alteration"
  Data Type Conversion4/1 -> Bus Creator/4  "IPM_LeftLeftLine_dy"
  Data Type Conversion5/1 -> Bus Creator/5  "IPM_LeftLeftLine_hor_curve"
  Data Type Conversion6/1 -> Bus Creator/6  "IPM_LeftLeftLine_yawangle"
  Data Type Conversion7/1 -> Bus Creator/7  "IPM_LeftLine_Color"
  Data Type Conversion8/1 -> Bus Creator/8  "IPM_LeftLine_Type"
  Data Type Conversion9/1 -> Bus Creator/9  "IPM_LineAssit_LeftLeftVisualization"
  Bus Creator/1 -> VR_ADCU_IPM_LeftLine_0x380FromOutData/1  "VR_ADCU_IPM_LeftLine_0x380FromOutData"
  VR_ADCU_IPM_LeftLine_0x380FromInData/1 -> CAN FD Unpack/1  "VR_ADCU_IPM_LeftLine_0x380FromInData"

== system ALL_JP360_DBW_V6_5_1103/MsgFromCAN/VR_ADCU_MsgFromCAN/VR_ADCU_IPM_LineHeader_0x631 ==
  VR_ADCU_IPM_LineHeader_0x631FromInData : Inport  OutDataTypeStr=Bus:CAN_FD_MESSAGE_BUS
  Bus Creator : BusCreator  Inputs=7  OutDataTypeStr=Bus:VR_ADCU_IPM_LineHeader_0x631  NonVirtualBus=on
  CAN FD Unpack : canfdmsglib/CAN FD Unpack  CANdbFile=HiFire_T360_P789_1R1V_Pri_Matrix_CAN_V2.3_20220810.dbc  MsgList=(none)  MsgName=IPM_LineHeader_0x631  ProtocolMode=CAN FD  MsgIDType=Standard (11-bit identifier)  MsgIdentifier=1585  MsgLength=20  SignalInfo={'IPM_LineHdr_State','5','3','BE','unsigned','Standard','0','1','0','0','7';'IPM_LineHeaderBlockCounter','85','11','BE','unsigned','Standard','0','1','0','0','2047';'IPM_LineHeader_Checksum','152','16','BE','unsigned','Standard','0','1','0','0','65535';'IPM_LineHeader_MsgCounter','136','4','BE','unsigned','Standard','0','1','0','0','15';'IPM_Line_TimeStampStatus','88','8','BE','unsigned','Standard','0','1','0','0','255';'IPM_Line_TimeStamp_Nsec','66','30','BE','unsigned','Standard','0','1','0','0','1073741823';'IPM_Line_TimeStamp_sec','32','32','BE','unsigned','Standard','0','1','0','0','4294967295'}  IDPort=off  TimestampPort=off  ErrorPort=off  RemotePort=off  LengthPort=off  StatusPort=off  BRSPort=off  ESIPort=off  DLCPort=off  ApplyMinMax=off
      settings: SourceProductBaseCode=ME,XP,VN  DataFormat=CANdb specified signals
  Data Type Conversion1 : DataTypeConversion  OutDataTypeStr=int8  SaturateOnIntegerOverflow=off  RndMeth=Floor
  Data Type Conversion2 : DataTypeConversion  OutDataTypeStr=int16  SaturateOnIntegerOverflow=off  RndMeth=Floor
  Data Type Conversion3 : DataTypeConversion  OutDataTypeStr=uint16  SaturateOnIntegerOverflow=off  RndMeth=Floor
  Data Type Conversion4 : DataTypeConversion  OutDataTypeStr=int8  SaturateOnIntegerOverflow=off  RndMeth=Floor
  Data Type Conversion5 : DataTypeConversion  OutDataTypeStr=uint8  SaturateOnIntegerOverflow=off  RndMeth=Floor
  Data Type Conversion6 : DataTypeConversion  OutDataTypeStr=int32  SaturateOnIntegerOverflow=off  RndMeth=Floor
  Data Type Conversion7 : DataTypeConversion  OutDataTypeStr=uint32  SaturateOnIntegerOverflow=off  RndMeth=Floor
  VR_ADCU_IPM_LineHeader_0x631FromOutData : Outport  OutDataTypeStr=Bus:VR_ADCU_IPM_LineHeader_0x631
  wires:
  CAN FD Unpack/1 -> Data Type Conversion1/1
  CAN FD Unpack/2 -> Data Type Conversion2/1
  CAN FD Unpack/3 -> Data Type Conversion3/1
  CAN FD Unpack/4 -> Data Type Conversion4/1
  CAN FD Unpack/5 -> Data Type Conversion5/1
  CAN FD Unpack/6 -> Data Type Conversion6/1
  CAN FD Unpack/7 -> Data Type Conversion7/1
  Data Type Conversion1/1 -> Bus Creator/1  "IPM_LineHdr_State"
  Data Type Conversion2/1 -> Bus Creator/2  "IPM_LineHeaderBlockCounter"
  Data Type Conversion3/1 -> Bus Creator/3  "IPM_LineHeader_Checksum"
  Data Type Conversion4/1 -> Bus Creator/4  "IPM_LineHeader_MsgCounter"
  Data Type Conversion5/1 -> Bus Creator/5  "IPM_Line_TimeStampStatus"
  Data Type Conversion6/1 -> Bus Creator/6  "IPM_Line_TimeStamp_Nsec"
  Data Type Conversion7/1 -> Bus Creator/7  "IPM_Line_TimeStamp_sec"
  Bus Creator/1 -> VR_ADCU_IPM_LineHeader_0x631FromOutData/1  "VR_ADCU_IPM_LineHeader_0x631FromOutData"
  VR_ADCU_IPM_LineHeader_0x631FromInData/1 -> CAN FD Unpack/1  "VR_ADCU_IPM_LineHeader_0x631FromInData"
